simulink model "Crazyflie_velosity_control_PID"  (R2020b)
settings: Solver=VariableStepAuto  StartTime=0.0  StopTime=5  RelTol=1e-3
libraries: pid_lib x3
settings Model: Creator=kt012  LastModifiedBy=kt012

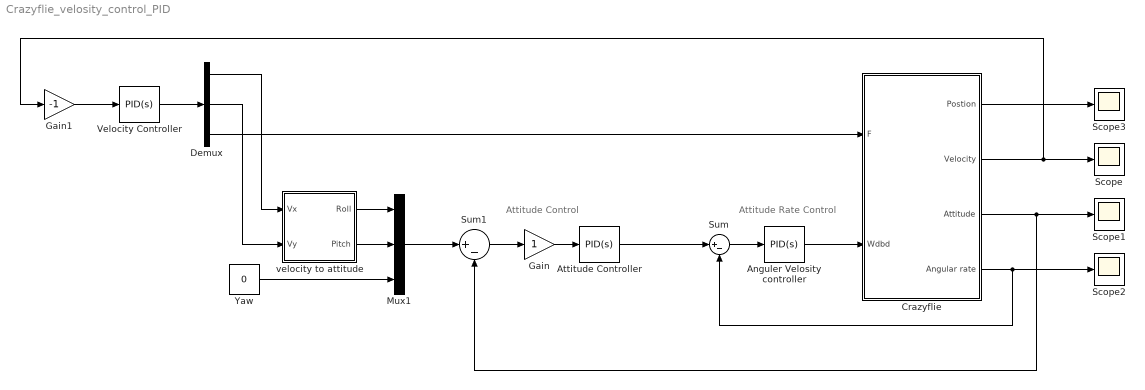
== system Crazyflie_velosity_control_PID ==
  note: Attitude Control
  note: Attitude Rate Control
  Anguler Velosity controller : pid_lib/PID Controller  Controller=PID  Form=Parallel  TimeDomain=Continuous-time  UseExternalTs=off  SampleTime=-1  IntegratorMethod=Forward Euler  FilterMethod=Forward Euler  ControllerParametersSource=internal  P=250 * 180 / 3.14  I=500 * 180 / 3.14  D=2.5 * 180 / 3.14  UseFilter=on  N=100  TunerSelectOption=Transfer Function Based (PID Tuner App)  InitialConditionSource=internal  InitialConditionForIntegrator=0  InitialConditionForFilter=0  DifferentiatorICPrevScaledInput=0  ExternalReset=none  TrackingMode=off  Kt=1  LimitOutput=off  SatLimitsSource=internal  UpperSaturationLimit=inf  LowerSaturationLimit=-inf  LinearizeAsGain=on  AntiWindupMode=none  Kb=1  POutMin=[]  POutMax=[]  IOutMin=[]  IOutMax=[]  DOutMin=[]  DOutMax=[]  NOutMin=[]  NOutMax=[]  SumOutMin=[]  SumOutMax=[]  SaturationOutMin=[]  SaturationOutMax=[]  PParamMin=[]  PParamMax=[]  IParamMin=[]  IParamMax=[]  DParamMin=[]  DParamMax=[]  NParamMin=[]  NParamMax=[]  KbParamMin=[]  KbParamMax=[]  KtParamMin=[]  KtParamMax=[]  KbOutMin=[]  KbOutMax=[]  KtOutMin=[]  KtOutMax=[]  IntegratorOutMin=[]  IntegratorOutMax=[]  FilterOutMin=[]  FilterOutMax=[]  SumI1OutMin=[]  SumI1OutMax=[]  SumI2OutMin=[]  SumI2OutMax=[]  SumI3OutMin=[]  SumI3OutMax=[]  SumI4OutMin=[]  SumI4OutMax=[]  SumDOutMin=[]  SumDOutMax=[]  DifferentiatorOutMin=[]  DifferentiatorOutMax=[]  FilterDiffOutCoefMin=[]  FilterDiffOutCoefMax=[]  ReciprocalOutMin=[]  ReciprocalOutMax=[]  SumDenOutMin=[]  SumDenOutMax=[]  SumNumOutMin=[]  SumNumOutMax=[]  DivideOutMin=[]  DivideOutMax=[]  UdiffTsProdOutMin=[]  UdiffTsProdOutMax=[]  NTsProdOutMin=[]  NTsProdOutMax=[]  UintegralTsProdOutMin=[]  UintegralTsProdOutMax=[]  UngainTsProdOutMin=[]  UngainTsProdOutMax=[]  IntegratorContinuousStateAttributes=''  IntegratorStateMustResolveToSignalObject=off  IntegratorRTWStateStorageClass=Auto  FilterContinuousStateAttributes=''  FilterStateMustResolveToSignalObject=off  FilterRTWStateStorageClass=Auto  ParallelPVariant=InternalParameters  IdealPVariant=Disabled  IVariant=InternalParameters  DVariant=InternalParameters  IntegratorVariant=Continuous  SatVariant=Disabled  AWVariant=Passthrough  PCopyVariant=Disabled  TRVariant=Disabled  FdbkBlocksVariant=Forward  IdealPFdbkVariant=Disabled  SatFdbkVariant=Disabled  DerivativeFilterVariant=ContFilter  NVariant=InternalParameters  NCopyVariant=Disabled  FilterICVariant=InternalICsFilter  IntegratorICVariant=InternalICs  ExternalResetVariant=Disabled  TRSumVariant=Passthrough  SumFdbkVariant=Disabled  SumVariant=Sum_PID  TsampFilterVariant=InternalTs  TsampNgainVariant=Passthrough  TsampIntegralVariant=Passthrough  ExternalSaturationOutDataTypeStr=Inherit: Same as second input
  Attitude Controller : pid_lib/PID Controller  Controller=PID  Form=Parallel  TimeDomain=Continuous-time  UseExternalTs=off  SampleTime=-1  IntegratorMethod=Forward Euler  FilterMethod=Forward Euler  ControllerParametersSource=internal  P=6.0 * 180 / 3.14  I=3.0 * 180 / 3.14  D=25  UseFilter=on  N=100  TunerSelectOption=Transfer Function Based (PID Tuner App)  InitialConditionSource=internal  InitialConditionForIntegrator=0  InitialConditionForFilter=0  DifferentiatorICPrevScaledInput=0  ExternalReset=none  TrackingMode=off  Kt=1  LimitOutput=off  SatLimitsSource=internal  UpperSaturationLimit=inf  LowerSaturationLimit=-inf  LinearizeAsGain=on  AntiWindupMode=none  Kb=1  POutMin=[]  POutMax=[]  IOutMin=[]  IOutMax=[]  DOutMin=[]  DOutMax=[]  NOutMin=[]  NOutMax=[]  SumOutMin=[]  SumOutMax=[]  SaturationOutMin=[]  SaturationOutMax=[]  PParamMin=[]  PParamMax=[]  IParamMin=[]  IParamMax=[]  DParamMin=[]  DParamMax=[]  NParamMin=[]  NParamMax=[]  KbParamMin=[]  KbParamMax=[]  KtParamMin=[]  KtParamMax=[]  KbOutMin=[]  KbOutMax=[]  KtOutMin=[]  KtOutMax=[]  IntegratorOutMin=[]  IntegratorOutMax=[]  FilterOutMin=[]  FilterOutMax=[]  SumI1OutMin=[]  SumI1OutMax=[]  SumI2OutMin=[]  SumI2OutMax=[]  SumI3OutMin=[]  SumI3OutMax=[]  SumI4OutMin=[]  SumI4OutMax=[]  SumDOutMin=[]  SumDOutMax=[]  DifferentiatorOutMin=[]  DifferentiatorOutMax=[]  FilterDiffOutCoefMin=[]  FilterDiffOutCoefMax=[]  ReciprocalOutMin=[]  ReciprocalOutMax=[]  SumDenOutMin=[]  SumDenOutMax=[]  SumNumOutMin=[]  SumNumOutMax=[]  DivideOutMin=[]  DivideOutMax=[]  UdiffTsProdOutMin=[]  UdiffTsProdOutMax=[]  NTsProdOutMin=[]  NTsProdOutMax=[]  UintegralTsProdOutMin=[]  UintegralTsProdOutMax=[]  UngainTsProdOutMin=[]  UngainTsProdOutMax=[]  IntegratorContinuousStateAttributes=''  IntegratorStateMustResolveToSignalObject=off  IntegratorRTWStateStorageClass=Auto  FilterContinuousStateAttributes=''  FilterStateMustResolveToSignalObject=off  FilterRTWStateStorageClass=Auto  ParallelPVariant=InternalParameters  IdealPVariant=Disabled  IVariant=InternalParameters  DVariant=InternalParameters  IntegratorVariant=Continuous  SatVariant=Disabled  AWVariant=Passthrough  PCopyVariant=Disabled  TRVariant=Disabled  FdbkBlocksVariant=Forward  IdealPFdbkVariant=Disabled  SatFdbkVariant=Disabled  DerivativeFilterVariant=ContFilter  NVariant=InternalParameters  NCopyVariant=Disabled  FilterICVariant=InternalICsFilter  IntegratorICVariant=InternalICs  ExternalResetVariant=Disabled  TRSumVariant=Passthrough  SumFdbkVariant=Disabled  SumVariant=Sum_PID  TsampFilterVariant=InternalTs  TsampNgainVariant=Passthrough  TsampIntegralVariant=Passthrough  ExternalSaturationOutDataTypeStr=Inherit: Same as second input
  Crazyflie : Subsystem
  Demux : Demux  Outputs=3
  Gain : Gain
  Gain1 : Gain  Gain=-1
  Mux1 : Mux  Inputs=3
  Scope{,1..3} (4 alike) : Scope
  Sum : Sum  Inputs=|+-
  Sum1 : Sum  Inputs=|+-
  Velocity Controller : pid_lib/PID Controller  Controller=PID  Form=Parallel  TimeDomain=Continuous-time  UseExternalTs=off  SampleTime=-1  IntegratorMethod=Forward Euler  FilterMethod=Forward Euler  ControllerParametersSource=internal  P=25  I=10  D=0  UseFilter=on  N=100  TunerSelectOption=Transfer Function Based (PID Tuner App)  InitialConditionSource=internal  InitialConditionForIntegrator=0  InitialConditionForFilter=0  DifferentiatorICPrevScaledInput=0  ExternalReset=none  TrackingMode=off  Kt=1  LimitOutput=off  SatLimitsSource=internal  UpperSaturationLimit=inf  LowerSaturationLimit=-inf  LinearizeAsGain=on  AntiWindupMode=none  Kb=1  POutMin=[]  POutMax=[]  IOutMin=[]  IOutMax=[]  DOutMin=[]  DOutMax=[]  NOutMin=[]  NOutMax=[]  SumOutMin=[]  SumOutMax=[]  SaturationOutMin=[]  SaturationOutMax=[]  PParamMin=[]  PParamMax=[]  IParamMin=[]  IParamMax=[]  DParamMin=[]  DParamMax=[]  NParamMin=[]  NParamMax=[]  KbParamMin=[]  KbParamMax=[]  KtParamMin=[]  KtParamMax=[]  KbOutMin=[]  KbOutMax=[]  KtOutMin=[]  KtOutMax=[]  IntegratorOutMin=[]  IntegratorOutMax=[]  FilterOutMin=[]  FilterOutMax=[]  SumI1OutMin=[]  SumI1OutMax=[]  SumI2OutMin=[]  SumI2OutMax=[]  SumI3OutMin=[]  SumI3OutMax=[]  SumI4OutMin=[]  SumI4OutMax=[]  SumDOutMin=[]  SumDOutMax=[]  DifferentiatorOutMin=[]  DifferentiatorOutMax=[]  FilterDiffOutCoefMin=[]  FilterDiffOutCoefMax=[]  ReciprocalOutMin=[]  ReciprocalOutMax=[]  SumDenOutMin=[]  SumDenOutMax=[]  SumNumOutMin=[]  SumNumOutMax=[]  DivideOutMin=[]  DivideOutMax=[]  UdiffTsProdOutMin=[]  UdiffTsProdOutMax=[]  NTsProdOutMin=[]  NTsProdOutMax=[]  UintegralTsProdOutMin=[]  UintegralTsProdOutMax=[]  UngainTsProdOutMin=[]  UngainTsProdOutMax=[]  IntegratorContinuousStateAttributes=''  IntegratorStateMustResolveToSignalObject=off  IntegratorRTWStateStorageClass=Auto  FilterContinuousStateAttributes=''  FilterStateMustResolveToSignalObject=off  FilterRTWStateStorageClass=Auto  ParallelPVariant=InternalParameters  IdealPVariant=Disabled  IVariant=InternalParameters  DVariant=InternalParameters  IntegratorVariant=Continuous  SatVariant=Disabled  AWVariant=Passthrough  PCopyVariant=Disabled  TRVariant=Disabled  FdbkBlocksVariant=Forward  IdealPFdbkVariant=Disabled  SatFdbkVariant=Disabled  DerivativeFilterVariant=ContFilter  NVariant=InternalParameters  NCopyVariant=Disabled  FilterICVariant=InternalICsFilter  IntegratorICVariant=InternalICs  ExternalResetVariant=Disabled  TRSumVariant=Passthrough  SumFdbkVariant=Disabled  SumVariant=Sum_PID  TsampFilterVariant=InternalTs  TsampNgainVariant=Passthrough  TsampIntegralVariant=Passthrough  ExternalSaturationOutDataTypeStr=Inherit: Same as second input
  Yaw : Constant  Value=0
  velocity to attitude : MATLAB Function  TreatAsAtomicUnit=on
  wires:
  Sum/1 -> Anguler Velosity controller/1
  Attitude Controller/1 -> Sum/1
  Anguler Velosity controller/1 -> Crazyflie/2(Wdbd)
  Gain/1 -> Attitude Controller/1
  Crazyflie/1(Postion) -> Scope3/1
  Crazyflie/2(Velocity) -> Scope/1, Gain1/1
  Crazyflie/3(Attitude) -> Scope1/1, Sum1/2
  Crazyflie/4(Angular rate) -> Sum/2, Scope2/1
  Gain1/1 -> Velocity Controller/1
  Velocity Controller/1 -> Demux/1
  Demux/3 -> Crazyflie/1(F)
  Demux/2 -> velocity to attitude/2(Vy)
  Demux/1 -> velocity to attitude/1(Vx)
  velocity to attitude/1(Roll) -> Mux1/1
  velocity to attitude/2(Pitch) -> Mux1/2
  Yaw/1 -> Mux1/3
  Mux1/1 -> Sum1/1
  Sum1/1 -> Gain/1

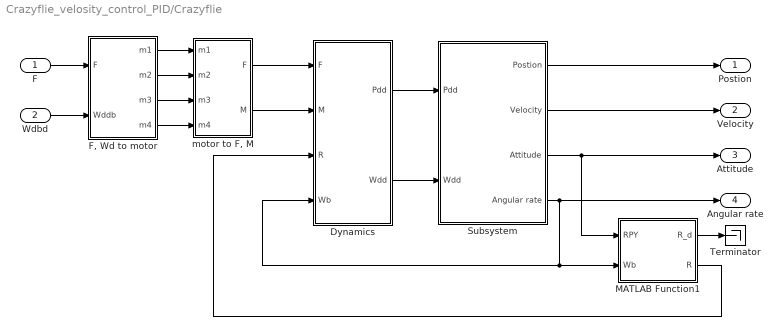
== system Crazyflie_velosity_control_PID/Crazyflie ==
  F : Inport
  Wdbd : Inport  Port=2
  Dynamics : MATLAB Function  TreatAsAtomicUnit=on
  "F, Wd to motor" : MATLAB Function  TreatAsAtomicUnit=on
  MATLAB Function1 : MATLAB Function  TreatAsAtomicUnit=on
  Subsystem : Subsystem
  Terminator : Terminator
  "motor to F, M" : MATLAB Function  TreatAsAtomicUnit=on
  Postion : Outport
  Velocity : Outport  Port=2
  Attitude : Outport  Port=3
  Angular rate : Outport  Port=4
  wires:
  "F, Wd to motor"/1(m1) -> "motor to F, M"/1(m1)
  Wdbd/1 -> "F, Wd to motor"/2(Wddb)
  "F, Wd to motor"/4(m4) -> "motor to F, M"/4(m4)
  "F, Wd to motor"/2(m2) -> "motor to F, M"/2(m2)
  "F, Wd to motor"/3(m3) -> "motor to F, M"/3(m3)
  Dynamics/2(Wdd) -> Subsystem/2(Wdd)
  "motor to F, M"/2(M) -> Dynamics/2(M)
  Subsystem/4(Angular rate) -> Angular rate/1, MATLAB Function1/2(Wb), Dynamics/4(Wb)
  "motor to F, M"/1(F) -> Dynamics/1(F)
  F/1 -> "F, Wd to motor"/1(F)
  Dynamics/1(Pdd) -> Subsystem/1(Pdd)
  Subsystem/3(Attitude) -> Attitude/1, MATLAB Function1/1(RPY)
  Subsystem/1(Postion) -> Postion/1
  Subsystem/2(Velocity) -> Velocity/1
  MATLAB Function1/2(R) -> Dynamics/3(R)
  MATLAB Function1/1(R_d) -> Terminator/1

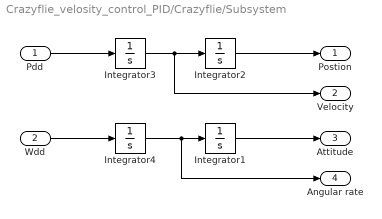
== system Crazyflie_velosity_control_PID/Crazyflie/Subsystem ==
  Pdd : Inport
  Wdd : Inport  Port=2
  Integrator1 : Integrator  InitialCondition=[0 0 0];
  Integrator2 : Integrator  InitialCondition=[0 0 0];
  Integrator3 : Integrator  InitialCondition=[1 0 0];
  Integrator4 : Integrator  InitialCondition=[0 0 0];
  Postion : Outport
  Velocity : Outport  Port=2
  Attitude : Outport  Port=3
  Angular rate : Outport  Port=4
  wires:
  Wdd/1 -> Integrator4/1
  Integrator4/1 -> Angular rate/1, Integrator1/1
  Integrator1/1 -> Attitude/1
  Pdd/1 -> Integrator3/1
  Integrator3/1 -> Integrator2/1, Velocity/1
  Integrator2/1 -> Postion/1

== matlab function Crazyflie_velosity_control_PID/Crazyflie/F, Wd to motor ==
  data: F input; Wddb input; m1 output; m2 output; m3 output; m4 output
function [m1, m2, m3, m4]= fcn(F, Wddb)

% F [16bit] Wddb [16bit]
F = F * 1000 + 32000;

r = min(max(-32000, Wddb(1)), 32000)/2;
p = min(max(-32000, Wddb(2)), 32000)/2;
y = min(max(-32000, Wddb(3)), 32000);

m1 = min(max(0,F - r - p + y), 2^16);
m2 = min(max(0,F - r + p - y), 2^16);
m3 = min(max(0,F + r + p + y), 2^16);
m4 = min(max(0,F + r - p - y), 2^16);

% formation +
% r = min(max(-32000, Wddb(1)), 32000);
% p = min(max(-32000, Wddb(2)), 32000);
% y = min(max(-32000, Wddb(3)), 32000);
% m1 = min(max(0, + p + y), 2^16);
% m2 = min(max(0, - r - y), 2^16);
% m3 = min(max(0, - p + y), 2^16);
% m4 = min(max(0, + r - y), 2^16);

%         ^y
%         |
%         |
%   m3          m4
%
%                    ------>x
%
%   m2          m1

== matlab function Crazyflie_velosity_control_PID/Crazyflie/MATLAB Function1 ==
  data: RPY input; Wb input; R_d output; R output
function [R_d, R]= fcn(RPY, Wb)
% 角速度 Vee演算
Wb = [ 0     -Wb(3)   Wb(2);
       Wb(3)  0       -Wb(1);
      -Wb(2)  Wb(1)   0   ];

% RPYから回転行列計算
roll = RPY(1);
pitch= RPY(2);
yaw = RPY(3);

R3 = [ cos(yaw) -sin(yaw) 0; sin(yaw) cos(yaw) 0; 0 0 1];              % ヨー角
R2 = [ cos(pitch) 0 -sin(pitch); 0 1 0; sin(pitch) 0 cos(pitch) ];     % ピッチ角
R1 = [ 1 0 0; 0 cos(roll) -sin(roll); 0 sin(roll) cos(roll)];          % ロール角

R = R1 * R2 * R3;   % 回転行列（ボディー　-> ワールド）

R_d = R * Wb;       % 微小時間の回転行列

== matlab function Crazyflie_velosity_control_PID/velocity to attitude ==
  data: Vx input; Roll output; Pitch output; Vy input
function [Roll, Pitch]= fcn(Vx, Vy)

Roll = -Vy * 3.14 / 180;
Pitch = -Vx * 3.14 / 180;

== matlab function Crazyflie_velosity_control_PID/Crazyflie/motor to F, M ==
  data: F output; m1 input; m2 input; M output; m3 input; m4 input
function [F, M] = func(m1, m2, m3, m4)

% F [16bit] Wddb [16bit]

Armlength = 0.092/2;
m1 = 2.130295 * 10^(-11) * m1^2 + 1.032633 * 10^(-6) * m1 + 5.484560 * 10^(-4);
m2 = 2.130295 * 10^(-11) * m2^2 + 1.032633 * 10^(-6) * m2 + 5.484560 * 10^(-4);
m3 = 2.130295 * 10^(-11) * m3^2 + 1.032633 * 10^(-6) * m3 + 5.484560 * 10^(-4);
m4 = 2.130295 * 10^(-11) * m4^2 + 1.032633 * 10^(-6) * m4 + 5.484560 * 10^(-4);

% calculate thrust
F = m1 + m2 + m3 + m4;

% calculate moment formation X
M1 = Armlength / sqrt(2) * (m3 + m4 - m1 - m2);
M2 = -Armlength / sqrt(2) * (-m3 - m2 + m1 + m4);

% calculate moment formation + 
% M1 = Armlength  * (m4 - m2);
% M2 = Armlength * (m1 - m3);

M3 = m1 + m3 - m2 - m4;

M = [M1 M2 M3]';

== matlab function Crazyflie_velosity_control_PID/Crazyflie/Dynamics ==
  data: Pdd output; F input; M input; R input; Wb input; Wdd output
function [Pdd,Wdd] = fcn(F, M, R, Wb)
m = 0.028;
e3 = [0 0 1]';
g = 9.8;
% % crazyflie
I = [16.571710 0.830806 0.718277;
     0.830806 16.655602 1.800197;
     0.718277 1.800197 29.261652] * 10^(-6);      % crazyflieの慣性モーメント（kg・m^2）
I = [1 0 0;
     0 1 0;
     0 0 1] * 10^(-6);
% 機体上向き加速度
Pdd = (R*F*e3 - m*g*e3)/m;

% 各加速度計算（ボディー座標系）
Wdd = pinv(I)*(M - cross(Wb, I * Wb));
